simulink library "uav_library"  (R2016a)
settings: Solver=ode45  StartTime=0.0  StopTime=10.0  RelTol=1e-3
libraries: uav_library x51, aerolibutil x5, simulink x2, aerolibtransform2 x1
settings Model: Creator=Maxence  LastModifiedBy=Maxence
settings DataIOCC: LimitDataPoints=on
settings DebuggingCC: AllowSymbolicDim=off

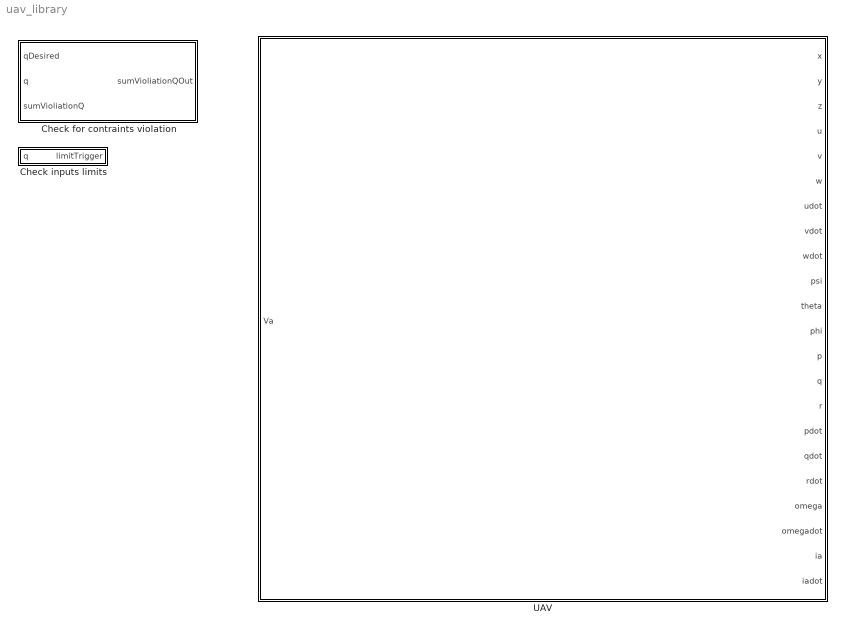
== system uav_library ==
  Check for contraints violation : Subsystem  mask{violationFactor=5, lowerQTol=0, upperQTol=0, currentTimeThreshold=0}
      mask prompts: violationFactor "Violation factor"; lowerQTol "Lower tolerance"; upperQTol "Upper tolerance"; currentTimeThreshold "Time threshold"
  Check inputs limits : Subsystem  mask{qMin=-1, qMax=1}
      mask prompts: qMin "Min value"; qMax "Max value"
  UAV : Subsystem  mask{g=9.80665, activateMast=on, config=X4, nMotors=4, m=0.312, I=[4.856e-3,0,0;0,4.856e-3,0;0,0,8.801e-3], PP=[0.16,0.16,-0.16,-0.16;0.16,-0.16,-0.16,0.16;0,0,0,0], Ra=0.5033*ones(4,1), La=1e-3*ones(4,1), ke=7.8e-3*ones(4,1), km=3.7e-3*ones(4,1), kD=1.140e-7*ones(4,1), Jm=3.357e-5*ones(4,1), Bm=1.23e-6*ones(4,1), kT=2.980e-6*ones(4,1), VaMin=0, VaMax=12, omegaInitial=zeros(4,1), omegaDelay=zeros(4,1), iaInitial=zeros(4,1), iaDelay=zeros(4,1), vPtInitial=zeros(3,1), vPtDelay=zeros(3,1), xPInitial=zeros(3,1), xPDelay=zeros(3,1), omegabtInitial=zeros(3,1), omegabtDelay=zeros(3,1), eulerZYXInitial=zeros(3,1), eulerZYXDelay=zeros(3,1)}
      mask prompts: g "Gravity (m/s^2)"; activateMast "Activate mask"; config "Configuration"; nMotors "Number of motors"; m "UAV mass (m) (kg)"; I "UAV Inertia tensor (I) (kg.m^2)"; PP "Motors position (PP) (m)"; Ra "Electrical resistance (Ra) (Ohm)"; La "Electrical inductance (La) (H)"; ke "Electromotive force constant (ke) (V/rad/s)"; km "Torque constant (km) (N.m/A)"; kD "Propeller drag parameter (kD) (N.m/rad^2/s^2)"; Jm "Rotor and propeller inertia (Jm) (kg*m^2)"; Bm "Viscous friction coefficient (Bm) (N.m/rad/s)"; kT "Propeller thrust coefficient (kT) (N/rad^2/s^2)"; VaMin "Voltage min (V)"; VaMax "Voltage max (V)"; omegaInitial "Angular velocity (rad/s)"; omegaDelay "Angular velocity delay (s)"; iaInitial "Current (A)"; iaDelay "Current delay (s)"; vPtInitial "Velocity (u, v, w) (m/s)"; vPtDelay "Velocity delay (u, v, w) (s)"; xPInitial "Position in tangent NED (m)"; xPDelay "Position in tangent NED delay (s)"; omegabtInitial "Angular rates (p, q, r) (rad/s)"; omegabtDelay "Angular rates delay (p, q, r) (s)"; eulerZYXInitial "Yaw, pitch, roll (psi, theta, phi) (rad)"; eulerZYXDelay "Yaw, pitch, roll delay (psi, theta, phi) (s)"
      mask TypeOptions config: X4 | I4 | X6 | I6 | I8 | V8
      mask Display:
      | if activateMast
      |     config = get_param(gcb,'config');
      |     position = get_param(gcb,'Position');
      |     width = abs(position(3) - position(1));
      |     height = abs(position(2) - position(4));
      |     width_ = width/1.8;
      |     if config == 'X4'
      |         height_ = width_*(654/643);
      |         posX = width/2 - width_/2;
      |         posY = height/2 - height_/2;
      |         image(imread('simulink_masks/Drone_Config_X4.jpg'),[posX,posY,width_,height_]) %
      |     elseif config == 'I4'
      |         height_ = width_*(832/850);
      |         posX = width/2 - width_/2;
      |         posY = height/2 - height_/2;
      |         image(imread('simulink_masks/Drone_Config_I4.jpg'),[posX,posY,width_,height_])
      |     elseif config == 'X6'
      |         height_ = width_*(759/811);
      |         posX = width/2 - width_/2;
      |         posY = height/2 - height_/2;
      |         image(imread('simulink_masks/Drone_Config_X6.jpg'),[posX,posY,width_,height_])
      |     elseif config == 'I6'
      |         height_ = width_*(812/732);
      |         posX = width/2 - width_/2;
      |         posY = height/2 - height_/2;
      |         image(imread('simulink_masks/Drone_Config_I6.jpg'),[posX,posY,width_,height_])
      |     elseif config == 'I8'
      |         height_ = width_*(827/809);
      |         posX = width/2 - width_/2;
      |         posY = height/2 - height_/2;
      |         image(imread('simulink_masks/Drone_Config_I8.jpg'),[posX,posY,width_,height_])
      |     elseif config == 'V8'
      |         height_ = width_*(806/784);
      |         posX = width/2 - width_/2;
      |         posY = height/2 - height_/2;
      |         image(imread('simulink_masks/Drone_Config_V8.jpg'),[posX,posY,width_,height_])
      |     end
      | end
      | 
      | % Ports label
      | port_label('input', 1, 'Va (V)')
      | port_label('output', 1, 'x (m)')
      | port_label('output', 2, 'y (m)')
      | port_label('output', 3, 'z (m)')
      | port_label('output', 4, 'u (m/s)')
      | port_label('output', 5, 'v (m/s)')
      | port_label('output', 6, 'w (m/s)')
      | port_label('output', 7, 'du/dt (m/s^2)')
      | port_label('output', 8, 'dv/dt (m/s^2)')
      | port_label('output', 9, 'dw/dt (m/s^2)')
      | port_label('output', 10, 'psi (rad)')
      | port_label('output', 11, 'theta (rad)')
      | port_label('output', 12, 'phi (rad)')
      | port_label('output', 13, 'p (rad/s)')
      | port_label('output', 14, 'q (rad/s)')
      | port_label('output', 15, 'r (rad/s)')
      | port_label('output', 16, 'dp/dt (rad/s^2)')
      | port_label('output', 17, 'dq/dt (rad/s^2)')
      | port_label('output', 18, 'dr/dt (rad/s^2)')
      | port_label('output', 19, 'omega (rad/s)')
      | port_label('output', 20, 'domega/dt (rad/s^2)')
      | port_label('output', 21, 'ia (A)')
      | port_label('output', 22, 'dia/dt (A/s)')

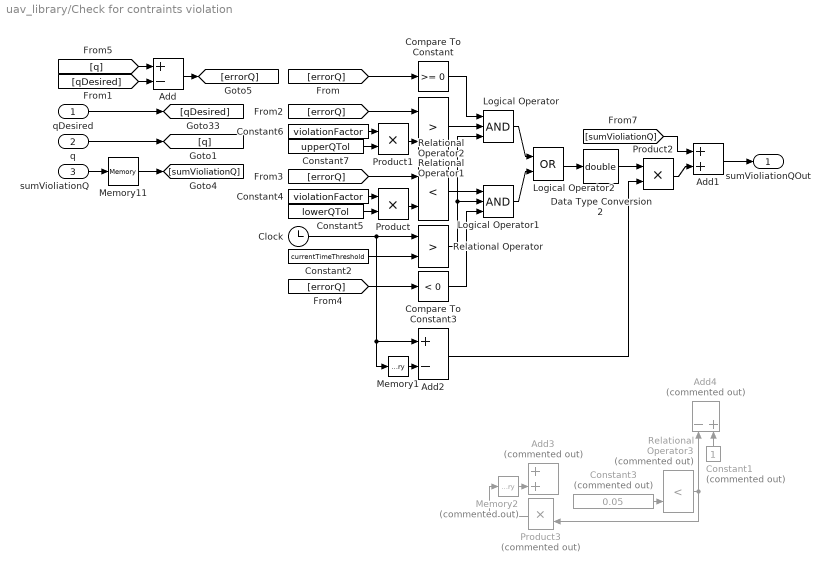
== system uav_library/Check for contraints violation ==
  qDesired : Inport
  q : Inport  Port=2
  sumVioliationQ : Inport  Port=3
  Add : Sum  Inputs=+-
  Add1 : Sum
  Add2 : Sum  Inputs=+-
  Add3 : Sum  Commented=on
  Add4 : Sum  Commented=on  Inputs=-+
  Clock : Clock
  Compare To Constant : simulink/Logic and Bit Operations/Compare To Constant  relop=>=  const=0  OutDataTypeStr=boolean  ZeroCross=off
  Compare To Constant3 : simulink/Logic and Bit Operations/Compare To Constant  relop=<  const=0  OutDataTypeStr=boolean  ZeroCross=off
  Constant1 : Constant  Commented=on
  Constant2 : Constant  Value=currentTimeThreshold
  Constant3 : Constant  Commented=on  Value=0.05
  Constant4 : Constant  Value=violationFactor
  Constant5 : Constant  Value=lowerQTol
  Constant6 : Constant  Value=violationFactor
  Constant7 : Constant  Value=upperQTol
  Data Type Conversion2 : DataTypeConversion  OutDataTypeStr=double
  Logical Operator : Logic  Inputs=3  AllPortsSameDT=off  OutDataTypeStr=boolean
  Logical Operator1 : Logic  Inputs=3  AllPortsSameDT=off  OutDataTypeStr=boolean
  Logical Operator2 : Logic  Operator=OR  AllPortsSameDT=off  OutDataTypeStr=boolean
  Memory1 : Memory
  Memory11 : Memory
  Memory2 : Memory  Commented=on
  Product : Product
  Product1 : Product
  Product2 : Product
  Product3 : Product  Commented=on
  Relational Operator : RelationalOperator  Operator=>  OutDataTypeStr=boolean  ZeroCross=off
  Relational Operator1 : RelationalOperator  Operator=>  OutDataTypeStr=boolean  ZeroCross=off
  Relational Operator2 : RelationalOperator  Operator=<  OutDataTypeStr=boolean  ZeroCross=off
  Relational Operator3 : RelationalOperator  Commented=on  Operator=<  OutDataTypeStr=boolean  ZeroCross=off
  sumVioliationQOut : Outport
  wires:
  qDesired/1 -> [qDesired]
  q/1 -> [q]
  sumVioliationQ/1 -> Memory11/1
  [q] -> Add/1
  [qDesired] -> Add/2
  Add/1 -> [errorQ]
  [errorQ] -> Compare To Constant/1
  Constant2/1 -> Relational Operator/2
  Constant4/1 -> Product/1
  Constant5/1 -> Product/2
  Constant6/1 -> Product1/1
  Constant7/1 -> Product1/2
  [errorQ] -> Relational Operator1/1
  Product1/1 -> Relational Operator1/2
  [errorQ] -> Relational Operator2/1
  Product/1 -> Relational Operator2/2
  Relational Operator2/1 -> Logical Operator1/1
  Relational Operator1/1 -> Logical Operator/2
  Relational Operator/1 -> Logical Operator/3, Logical Operator1/2
  [errorQ] -> Compare To Constant3/1
  Compare To Constant3/1 -> Logical Operator1/3
  Compare To Constant/1 -> Logical Operator/1
  Add1/1 -> sumVioliationQOut/1
  [sumVioliationQ] -> Add1/1
  Logical Operator/1 -> Logical Operator2/1
  Logical Operator1/1 -> Logical Operator2/2
  Logical Operator2/1 -> Data Type Conversion2/1
  Memory11/1 -> [sumVioliationQ]
  Data Type Conversion2/1 -> Product2/1
  Product2/1 -> Add1/2
  Clock/1 -> Relational Operator/1, Memory1/1, Add2/1
  Memory1/1 -> Add2/2
  Add2/1 -> Product2/2
  Memory2/1 -> Add3/2
  Constant3/1 -> Relational Operator3/2
  Product3/1 -> Memory2/1
  Relational Operator3/1 -> Add4/1, Product3/2
  Constant1/1 -> Add4/2

== system uav_library/Check inputs limits ==
  q : Inport
  Constant5 : Constant  Value=qMin
  Constant6 : Constant  Value=qMax
  Data Type Conversion2 : DataTypeConversion  OutDataTypeStr=double
  Logical Operator2 : Logic  Operator=OR  AllPortsSameDT=off  OutDataTypeStr=boolean
  Relational Operator12 : RelationalOperator  Operator=<  OutDataTypeStr=boolean  ZeroCross=off
  Relational Operator13 : RelationalOperator  Operator=>  OutDataTypeStr=boolean  ZeroCross=off
  limitTrigger : Outport
  wires:
  Constant5/1 -> Relational Operator12/2
  Constant6/1 -> Relational Operator13/2
  q/1 -> Relational Operator13/1, Relational Operator12/1
  Relational Operator12/1 -> Logical Operator2/1
  Relational Operator13/1 -> Logical Operator2/2
  Logical Operator2/1 -> Data Type Conversion2/1
  Data Type Conversion2/1 -> limitTrigger/1

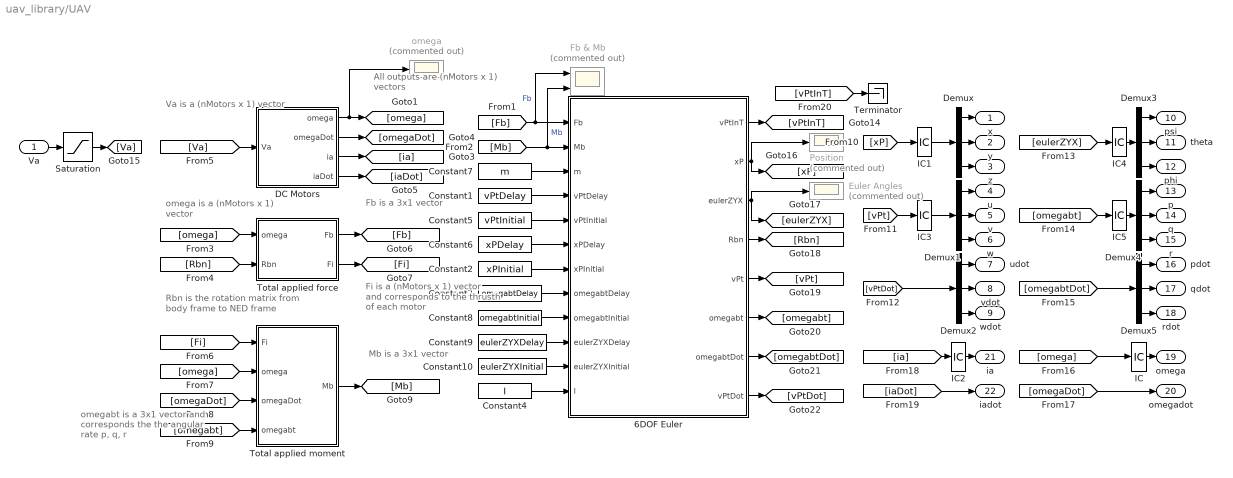
== system uav_library/UAV ==
  note: Va is a (nMotors x 1) vector
  note: All outputs are (nMotors x 1) vectors
  note: Rbn is the rotation matrix from body frame to NED frame
  note: omega is a (nMotors x 1) vector
  note: Fb is a 3x1 vector
  note: Fi is a (nMotors x 1) vector and corresponds to the thrusth of each motor
  note: Mb is a 3x1 vector
  note: omegabt is a 3x1 vector and corresponds the the angular rate p, q, r
  Va : Inport
  " omega" : Scope  Commented=on
  6DOF Euler : Subsystem
  Constant1 : Constant  Value=vPtDelay
  Constant10 : Constant  Value=eulerZYXInitial
  Constant2 : Constant  Value=xPInitial
  Constant3 : Constant  Value=omegabtDelay
  Constant4 : Constant  Value=I
  Constant5 : Constant  Value=vPtInitial
  Constant6 : Constant  Value=xPDelay
  Constant7 : Constant  Value=m
  Constant8 : Constant  Value=omegabtInitial
  Constant9 : Constant  Value=eulerZYXDelay
  DC Motors : Subsystem
  Demux{,1..5} (6 alike) : Demux  Outputs=3
  Euler Angles : Scope  Commented=on
  Fb & Mb : Scope  Commented=on  NumInputPorts=2
  IC : InitialCondition  Value=omegaInitial
  IC1 : InitialCondition  Value=xPInitial
  IC2 : InitialCondition  Value=iaInitial
  IC3 : InitialCondition  Value=vPtInitial
  IC4 : InitialCondition  Value=eulerZYXInitial
  IC5 : InitialCondition  Value=omegabtInitial
  Position : Scope  Commented=on
  Saturation : Saturate  UpperLimit=VaMax  LowerLimit=VaMin
  Terminator : Terminator
  Total applied force : Subsystem
  Total applied moment : Subsystem
  x : Outport
  y : Outport  Port=2
  z : Outport  Port=3
  u : Outport  Port=4
  v : Outport  Port=5
  w : Outport  Port=6
  udot : Outport  Port=7
  vdot : Outport  Port=8
  wdot : Outport  Port=9
  psi : Outport  Port=10
  theta : Outport  Port=11
  phi : Outport  Port=12
  p : Outport  Port=13
  q : Outport  Port=14
  r : Outport  Port=15
  pdot : Outport  Port=16
  qdot : Outport  Port=17
  rdot : Outport  Port=18
  omega : Outport  Port=19
  omegadot : Outport  Port=20
  ia : Outport  Port=21
  iadot : Outport  Port=22
  wires:
  DC Motors/1(omega) -> " omega"/1, [omega]
  DC Motors/3(ia) -> [ia]
  DC Motors/2(omegaDot) -> [omegaDot]
  DC Motors/4(iaDot) -> [iaDot]
  Total applied force/1(Fb) -> [Fb]
  [Fb] -> 6DOF Euler/1(Fb), Fb & Mb/1  "Fb"
  [Mb] -> 6DOF Euler/2(Mb), Fb & Mb/2  "Mb"
  [omega] -> Total applied force/1(omega)
  [Rbn] -> Total applied force/2(Rbn)
  Total applied force/2(Fi) -> [Fi]
  [Va] -> DC Motors/1(Va)
  [Fi] -> Total applied moment/1(Fi)
  [omega] -> Total applied moment/2(omega)
  [omegaDot] -> Total applied moment/3(omegaDot)
  [omegabt] -> Total applied moment/4(omegabt)
  Total applied moment/1(Mb) -> [Mb]
  6DOF Euler/1(vPtInT) -> [vPtInT]
  [xP] -> IC1/1
  Demux/1 -> x/1
  Demux/2 -> y/1
  Demux/3 -> z/1
  6DOF Euler/2(xP) -> Position/1, [xP]
  6DOF Euler/3(eulerZYX) -> Euler Angles/1, [eulerZYX]
  6DOF Euler/4(Rbn) -> [Rbn]
  6DOF Euler/5(vPt) -> [vPt]
  6DOF Euler/6(omegabt) -> [omegabt]
  6DOF Euler/7(omegabtDot) -> [omegabtDot]
  6DOF Euler/8(vPtDot) -> [vPtDot]
  Constant7/1 -> 6DOF Euler/3(m)
  Constant1/1 -> 6DOF Euler/4(vPtDelay)
  Constant4/1 -> 6DOF Euler/12(I)
  Constant5/1 -> 6DOF Euler/5(vPtInitial)
  Constant6/1 -> 6DOF Euler/6(xPDelay)
  Constant2/1 -> 6DOF Euler/7(xPInitial)
  Constant3/1 -> 6DOF Euler/8(omegabtDelay)
  Constant8/1 -> 6DOF Euler/9(omegabtInitial)
  Constant9/1 -> 6DOF Euler/10(eulerZYXDelay)
  Constant10/1 -> 6DOF Euler/11(eulerZYXInitial)
  Va/1 -> Saturation/1
  [vPt] -> IC3/1
  Demux1/1 -> u/1
  Demux1/2 -> v/1
  Demux1/3 -> w/1
  [vPtDot] -> Demux2/1
  Demux2/1 -> udot/1
  Demux2/2 -> vdot/1
  Demux2/3 -> wdot/1
  [eulerZYX] -> IC4/1
  Demux3/1 -> psi/1
  Demux3/2 -> theta/1
  Demux3/3 -> phi/1
  Demux4/1 -> p/1
  Demux4/2 -> q/1
  Demux4/3 -> r/1
  [omegabtDot] -> Demux5/1
  Demux5/1 -> pdot/1
  Demux5/2 -> qdot/1
  Demux5/3 -> rdot/1
  [omega] -> IC/1
  [ia] -> IC2/1
  Saturation/1 -> [Va]
  [vPtInT] -> Terminator/1
  IC/1 -> omega/1
  [omegaDot] -> omegadot/1
  IC2/1 -> ia/1
  [iaDot] -> iadot/1
  IC1/1 -> Demux/1
  IC3/1 -> Demux1/1
  IC4/1 -> Demux3/1
  [omegabt] -> IC5/1
  IC5/1 -> Demux4/1

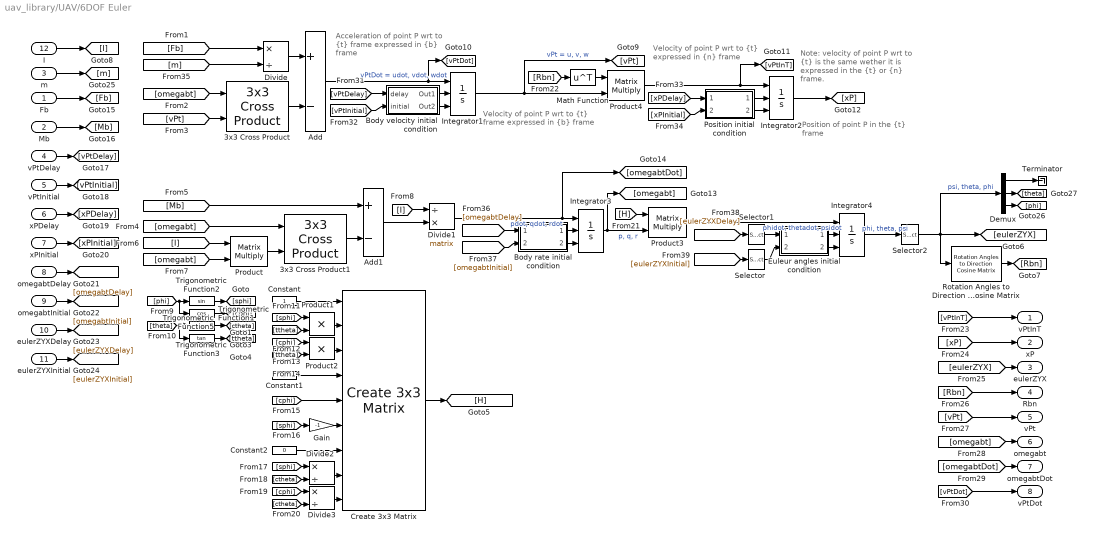
== system uav_library/UAV/6DOF Euler ==
  note: Acceleration of point P wrt to {t} frame expressed in {b} frame
  note: Velocity of point P wrt to {t} frame expressed in {b} frame
  note: Velocity of point P wrt to {t} expressed in {n} frame
  note: Position of point P in the {t} frame
  note: Note: velocity of point P wrt to {t} is the same wether it is expressed in the {t} or {n} frame.
  Fb : Inport
  Mb : Inport  Port=2
  m : Inport  Port=3
  vPtDelay : Inport  Port=4
  vPtInitial : Inport  Port=5
  xPDelay : Inport  Port=6
  xPInitial : Inport  Port=7
  omegabtDelay : Inport  Port=8
  omegabtInitial : Inport  Port=9
  eulerZYXDelay : Inport  Port=10
  eulerZYXInitial : Inport  Port=11
  I : Inport  Port=12
  3x3 Cross Product : aerolibutil/3x3 Cross Product
  3x3 Cross Product1 : aerolibutil/3x3 Cross Product
  Add : Sum  Inputs=+-
  Add1 : Sum  Inputs=+-
  Body rate initial condition : Subsystem
  Body velocity initial condition : Subsystem
  Constant : Constant
  Constant1 : Constant  Value=0
  Constant2 : Constant  Value=0
  Create 3x3 Matrix : aerolibutil/Create 3x3 Matrix
  Demux : Demux  Outputs=3
  Divide : Product  Inputs=*/
  Divide1 : Product  Inputs=/*  Multiplication=Matrix(*)
  Divide2 : Product  Inputs=*/
  Divide3 : Product  Inputs=*/
  Euleur angles initial condition : Subsystem
  Gain : Gain  Gain=-1
  Integrator1 : Integrator  ExternalReset=falling  InitialConditionSource=external
  Integrator2 : Integrator  ExternalReset=falling  InitialConditionSource=external
  Integrator3 : Integrator  ExternalReset=falling  InitialConditionSource=external
  Integrator4 : Integrator  ExternalReset=falling  InitialConditionSource=external  WrapState=on  WrappedStateUpperValue=[pi;pi/2;pi]  WrappedStateLowerValue=-[pi;pi/2;pi]
  Math Function : Math  Operator=transpose  SaturateOnIntegerOverflow=on
  Position initial condition : Subsystem
  Product : Product  Multiplication=Matrix(*)
  Product1 : Product
  Product2 : Product
  Product3 : Product  Multiplication=Matrix(*)
  Product4 : Product  Multiplication=Matrix(*)
  Rotation Angles to Direction Cosine Matrix : aerolibtransform2/Rotation Angles to Direction Cosine Matrix  rotationOrder=ZYX
  Selector : Selector  InputPortWidth=3  IndexOptions=Index vector (dialog)  Indices=[3 2 1]  OutputSizes=1
  Selector1 : Selector  InputPortWidth=3  IndexOptions=Index vector (dialog)  Indices=[3 2 1]  OutputSizes=1
  Selector2 : Selector  InputPortWidth=3  IndexOptions=Index vector (dialog)  Indices=[3 2 1]  OutputSizes=1
  Terminator : Terminator
  Trigonometric Function1 : Trigonometry  Operator=cos
  Trigonometric Function2 : Trigonometry
  Trigonometric Function3 : Trigonometry  Operator=cos
  Trigonometric Function5 : Trigonometry  Operator=tan
  vPtInT : Outport
  xP : Outport  Port=2
  eulerZYX : Outport  Port=3
  Rbn : Outport  Port=4
  vPt : Outport  Port=5
  omegabt : Outport  Port=6
  omegabtDot : Outport  Port=7
  vPtDot : Outport  Port=8
  wires:
  [omegabt] -> 3x3 Cross Product/1
  [vPt] -> 3x3 Cross Product/2
  [m] -> Divide/2
  [Fb] -> Divide/1
  Divide/1 -> Add/1
  3x3 Cross Product/1 -> Add/2
  Add/1 -> [vPtDot], Integrator1/1  "vPtDot = udot, vdot, wdot"
  Body velocity initial condition/1(Out1) -> Integrator1/2
  Body velocity initial condition/2(Out2) -> Integrator1/3
  [vPtDelay] -> Body velocity initial condition/1(delay)
  [vPtInitial] -> Body velocity initial condition/2(initial)
  Integrator1/1 -> Product4/2, [vPt]  "vPt = u, v, w"
  Position initial condition/1(Out1) -> Integrator2/2
  Position initial condition/2(Out2) -> Integrator2/3
  [xPDelay] -> Position initial condition/1(delay)
  [xPInitial] -> Position initial condition/2(initial)
  [omegabt] -> 3x3 Cross Product1/1
  [I] -> Product/1
  [omegabt] -> Product/2
  Product/1 -> 3x3 Cross Product1/2
  [Mb] -> Add1/1
  3x3 Cross Product1/1 -> Add1/2
  [I] -> Divide1/1
  Add1/1 -> Divide1/2
  Body rate initial condition/1(Out1) -> Integrator3/2
  Body rate initial condition/2(Out2) -> Integrator3/3
  [omegabtDelay] -> Body rate initial condition/1(delay)
  [omegabtInitial] -> Body rate initial condition/2(initial)
  Divide1/1 -> [omegabtDot], Integrator3/1  "pdot, qdot, rdot"
  Constant/1 -> Create 3x3 Matrix/1
  Constant1/1 -> Create 3x3 Matrix/4
  Constant2/1 -> Create 3x3 Matrix/7
  [phi] -> Trigonometric Function1/1, Trigonometric Function2/1
  Trigonometric Function2/1 -> [sphi]
  Trigonometric Function1/1 -> [cphi]
  [theta] -> Trigonometric Function5/1, Trigonometric Function3/1
  Trigonometric Function3/1 -> [ctheta]
  Trigonometric Function5/1 -> [ttheta]
  Product1/1 -> Create 3x3 Matrix/2
  [sphi] -> Product1/1
  [ttheta] -> Product1/2
  [cphi] -> Product2/1
  [ttheta] -> Product2/2
  Product2/1 -> Create 3x3 Matrix/3
  [cphi] -> Create 3x3 Matrix/5
  [sphi] -> Gain/1
  Gain/1 -> Create 3x3 Matrix/6
  Divide2/1 -> Create 3x3 Matrix/8
  Divide3/1 -> Create 3x3 Matrix/9
  [sphi] -> Divide2/1
  [ctheta] -> Divide2/2
  [cphi] -> Divide3/1
  [ctheta] -> Divide3/2
  Create 3x3 Matrix/1 -> [H]
  Integrator3/1 -> [omegabt], Product3/2  "p, q, r"
  [H] -> Product3/1
  Product3/1 -> Integrator4/1  "phidot, thetadot, psidot"
  Euleur angles initial condition/1(Out1) -> Integrator4/2
  Euleur angles initial condition/2(Out2) -> Integrator4/3
  Integrator4/1 -> Selector2/1  "phi, theta, psi"
  [eulerZYXInitial] -> Selector/1
  [eulerZYXDelay] -> Selector1/1
  Selector1/1 -> Euleur angles initial condition/1(delay)
  Selector/1 -> Euleur angles initial condition/2(initial)
  Selector2/1 -> Demux/1, Rotation Angles to Direction Cosine Matrix/1, [eulerZYX]  "psi, theta, phi"
  Rotation Angles to Direction Cosine Matrix/1 -> [Rbn]
  [Rbn] -> Math Function/1
  Product4/1 -> [vPtInT], Integrator2/1
  Integrator2/1 -> [xP]
  [vPtInT] -> vPtInT/1
  [xP] -> xP/1
  [eulerZYX] -> eulerZYX/1
  [Rbn] -> Rbn/1
  [vPt] -> vPt/1
  [omegabt] -> omegabt/1
  [omegabtDot] -> omegabtDot/1
  [vPtDot] -> vPtDot/1
  Fb/1 -> [Fb]
  Mb/1 -> [Mb]
  vPtDelay/1 -> [vPtDelay]
  vPtInitial/1 -> [vPtInitial]
  xPDelay/1 -> [xPDelay]
  xPInitial/1 -> [xPInitial]
  omegabtDelay/1 -> [omegabtDelay]
  omegabtInitial/1 -> [omegabtInitial]
  eulerZYXDelay/1 -> [eulerZYXDelay]
  eulerZYXInitial/1 -> [eulerZYXInitial]
  m/1 -> [m]
  Demux/2 -> [theta]
  Demux/3 -> [phi]
  Demux/1 -> Terminator/1
  I/1 -> [I]
  Math Function/1 -> Product4/1

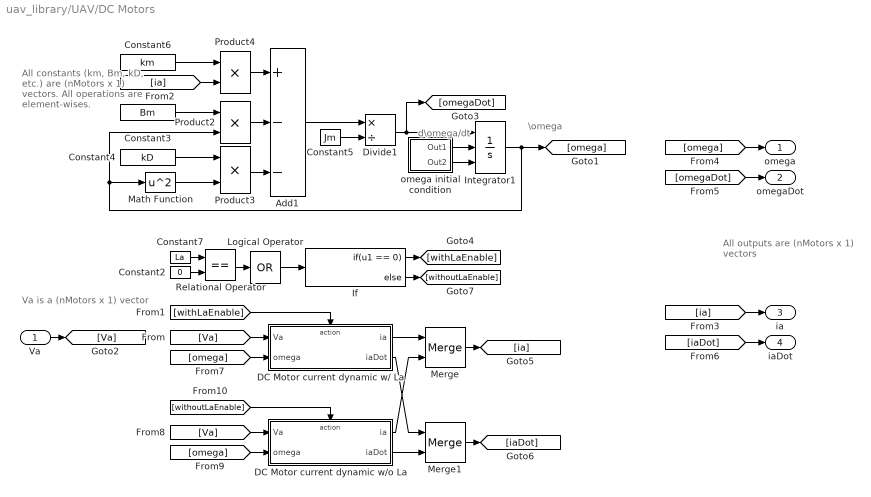
== system uav_library/UAV/DC Motors ==
  note: d\omega/dt
  note: \omega
  note: Va is a (nMotors x 1) vector
  note: All constants (km, Bm, kD, etc.) are (nMotors x 1) vectors.
      |
      | All operations are element-wises.
  note: All outputs are (nMotors x 1) vectors
  Va : Inport
  Add1 : Sum  Inputs=+--
  Constant2 : Constant  Value=0
  Constant3 : Constant  Value=Bm
  Constant4 : Constant  Value=kD
  Constant5 : Constant  Value=Jm
  Constant6 : Constant  Value=km
  Constant7 : Constant  Value=La
  DC Motor current dynamic w/ La : Subsystem  TreatAsAtomicUnit=on
  DC Motor current dynamic w/o La : Subsystem  TreatAsAtomicUnit=on
  Divide1 : Product  Inputs=*/
  If : If  IfExpression=u1 == 0
  Integrator1 : Integrator  ExternalReset=falling  InitialConditionSource=external
  Logical Operator : Logic  Operator=OR  Inputs=1  AllPortsSameDT=off  OutDataTypeStr=boolean
  Math Function : Math  Operator=square  SaturateOnIntegerOverflow=on
  Merge : Merge
  Merge1 : Merge
  Product2 : Product
  Product3 : Product
  Product4 : Product
  Relational Operator : RelationalOperator  Operator===  OutDataTypeStr=boolean
  omega initial condition : Subsystem
  omega : Outport
  omegaDot : Outport  Port=2
  ia : Outport  Port=3
  iaDot : Outport  Port=4
  wires:
  Product4/1 -> Add1/1
  Constant6/1 -> Product4/1
  [ia] -> Product4/2
  Product2/1 -> Add1/2
  Integrator1/1 -> [omega], Math Function/1, Product2/2
  Add1/1 -> Divide1/1
  Constant4/1 -> Product3/1
  Constant3/1 -> Product2/1
  Product3/1 -> Add1/3
  Constant5/1 -> Divide1/2
  Math Function/1 -> Product3/2
  Va/1 -> [Va]
  [ia] -> ia/1
  [omega] -> omega/1
  [omegaDot] -> omegaDot/1
  [iaDot] -> iaDot/1
  Divide1/1 -> [omegaDot], Integrator1/1
  omega initial condition/1(Out1) -> Integrator1/2
  omega initial condition/2(Out2) -> Integrator1/3
  Logical Operator/1 -> If/1
  DC Motor current dynamic w/o La/2(iaDot) -> Merge1/2
  [Va] -> DC Motor current dynamic w/ La/1(Va)
  DC Motor current dynamic w/ La/1(ia) -> Merge/1
  Merge/1 -> [ia]
  Merge1/1 -> [iaDot]
  [omega] -> DC Motor current dynamic w/ La/2(omega)
  [omega] -> DC Motor current dynamic w/o La/2(omega)
  [Va] -> DC Motor current dynamic w/o La/1(Va)
  If/1 -> [withLaEnable]
  If/2 -> [withoutLaEnable]
  [withLaEnable] -> DC Motor current dynamic w/ La/Action
  [withoutLaEnable] -> DC Motor current dynamic w/o La/Action
  DC Motor current dynamic w/ La/2(iaDot) -> Merge1/1
  DC Motor current dynamic w/o La/1(ia) -> Merge/2
  Relational Operator/1 -> Logical Operator/1
  Constant2/1 -> Relational Operator/2
  Constant7/1 -> Relational Operator/1

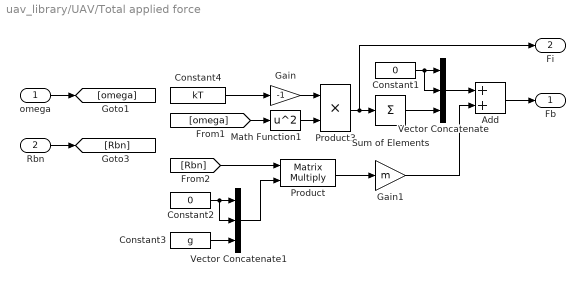
== system uav_library/UAV/Total applied force ==
  omega : Inport
  Rbn : Inport  Port=2
  Add : Sum
  Constant1 : Constant  Value=0
  Constant2 : Constant  Value=0
  Constant3 : Constant  Value=g
  Constant4 : Constant  Value=kT
  Gain : Gain  Gain=-1
  Gain1 : Gain  Gain=m
  Math Function1 : Math  Operator=square  SaturateOnIntegerOverflow=on
  Product : Product  Multiplication=Matrix(*)
  Product3 : Product
  Sum of Elements : Sum  Inputs=+
  Vector Concatenate : Concatenate  NumInputs=3
  Vector Concatenate1 : Concatenate  NumInputs=3
  Fb : Outport
  Fi : Outport  Port=2
  wires:
  Constant4/1 -> Gain/1
  Math Function1/1 -> Product3/2
  Product/1 -> Gain1/1
  Constant2/1 -> Vector Concatenate1/2, Vector Concatenate1/1
  Constant3/1 -> Vector Concatenate1/3
  Product3/1 -> Fi/1, Sum of Elements/1
  Add/1 -> Fb/1
  Vector Concatenate1/1 -> Product/2
  Sum of Elements/1 -> Vector Concatenate/3
  Gain/1 -> Product3/1
  Constant1/1 -> Vector Concatenate/2, Vector Concatenate/1
  Vector Concatenate/1 -> Add/1
  [omega] -> Math Function1/1
  omega/1 -> [omega]
  Rbn/1 -> [Rbn]
  [Rbn] -> Product/1
  Gain1/1 -> Add/2

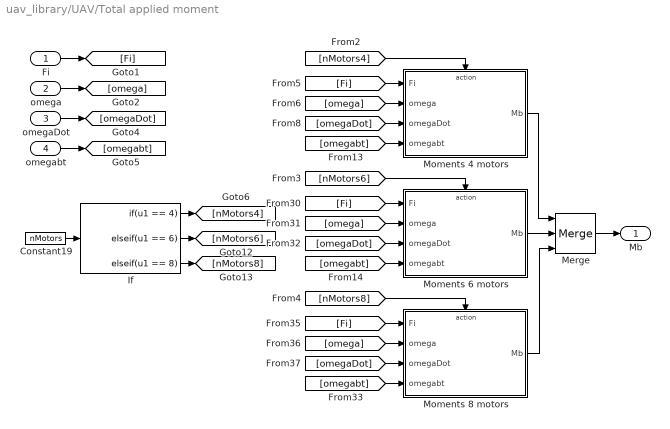
== system uav_library/UAV/Total applied moment ==
  Fi : Inport
  omega : Inport  Port=2
  omegaDot : Inport  Port=3
  omegabt : Inport  Port=4
  Constant19 : Constant  Value=nMotors
  If : If  IfExpression=u1 == 4  ElseIfExpressions=u1 == 6, u1 == 8  ShowElse=off
  Merge : Merge  Inputs=3
  Moments 4 motors : Subsystem  TreatAsAtomicUnit=on
  Moments 6 motors : Subsystem  TreatAsAtomicUnit=on
  Moments 8 motors : Subsystem  TreatAsAtomicUnit=on
  Mb : Outport
  wires:
  Fi/1 -> [Fi]
  omega/1 -> [omega]
  omegaDot/1 -> [omegaDot]
  omegabt/1 -> [omegabt]
  If/1 -> [nMotors4]
  If/2 -> [nMotors6]
  [nMotors4] -> Moments 4 motors/Action
  [nMotors6] -> Moments 6 motors/Action
  Constant19/1 -> If/1
  If/3 -> [nMotors8]
  [Fi] -> Moments 4 motors/1(Fi)
  [omega] -> Moments 4 motors/2(omega)
  [omegaDot] -> Moments 4 motors/3(omegaDot)
  [omegabt] -> Moments 4 motors/4(omegabt)
  [Fi] -> Moments 6 motors/1(Fi)
  [omega] -> Moments 6 motors/2(omega)
  [omegaDot] -> Moments 6 motors/3(omegaDot)
  [omegabt] -> Moments 6 motors/4(omegabt)
  [nMotors8] -> Moments 8 motors/Action
  [Fi] -> Moments 8 motors/1(Fi)
  [omega] -> Moments 8 motors/2(omega)
  [omegaDot] -> Moments 8 motors/3(omegaDot)
  [omegabt] -> Moments 8 motors/4(omegabt)
  Moments 6 motors/1(Mb) -> Merge/2
  Moments 4 motors/1(Mb) -> Merge/1
  Moments 8 motors/1(Mb) -> Merge/3
  Merge/1 -> Mb/1

== system uav_library/UAV/6DOF Euler/Body rate initial condition ==
  delay : Inport
  initial : Inport  Port=2
  Clock1 : Clock
  Sum4 : Sum  Inputs=|-+
  Triggered Subsystem2 : Subsystem  TreatAsAtomicUnit=on
  Out1 : Outport
  Out2 : Outport  Port=2
  wires:
  delay/1 -> Sum4/2
  Triggered Subsystem2/1(Out1) -> Out2/1
  Sum4/1 -> Out1/1, Triggered Subsystem2/Trigger
  Clock1/1 -> Sum4/1
  initial/1 -> Triggered Subsystem2/1(In1)

== system uav_library/UAV/6DOF Euler/Body velocity initial condition ==
  delay : Inport
  initial : Inport  Port=2
  Clock1 : Clock
  Sum4 : Sum  Inputs=|-+
  Triggered Subsystem2 : Subsystem  TreatAsAtomicUnit=on
  Out1 : Outport
  Out2 : Outport  Port=2
  wires:
  delay/1 -> Sum4/2
  Triggered Subsystem2/1(Out1) -> Out2/1
  Sum4/1 -> Out1/1, Triggered Subsystem2/Trigger
  Clock1/1 -> Sum4/1
  initial/1 -> Triggered Subsystem2/1(In1)

== system uav_library/UAV/6DOF Euler/Euleur angles initial condition ==
  delay : Inport
  initial : Inport  Port=2
  Clock1 : Clock
  Sum4 : Sum  Inputs=|-+
  Triggered Subsystem2 : Subsystem  TreatAsAtomicUnit=on
  Out1 : Outport
  Out2 : Outport  Port=2
  wires:
  delay/1 -> Sum4/2
  Triggered Subsystem2/1(Out1) -> Out2/1
  Sum4/1 -> Out1/1, Triggered Subsystem2/Trigger
  Clock1/1 -> Sum4/1
  initial/1 -> Triggered Subsystem2/1(In1)

== system uav_library/UAV/6DOF Euler/Position initial condition ==
  delay : Inport
  initial : Inport  Port=2
  Clock1 : Clock
  Sum4 : Sum  Inputs=|-+
  Triggered Subsystem2 : Subsystem  TreatAsAtomicUnit=on
  Out1 : Outport
  Out2 : Outport  Port=2
  wires:
  initial/1 -> Triggered Subsystem2/1(In1)
  Clock1/1 -> Sum4/1
  Sum4/1 -> Triggered Subsystem2/Trigger, Out1/1
  Triggered Subsystem2/1(Out1) -> Out2/1
  delay/1 -> Sum4/2

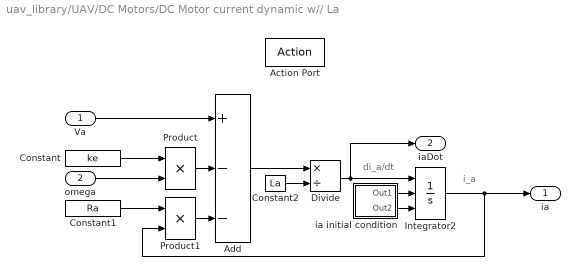
== system uav_library/UAV/DC Motors/DC Motor current dynamic w// La ==
  note: di_a/dt
  note: i_a
  Va : Inport
  omega : Inport  Port=2
  Action Port : ActionPort
  Add : Sum  Inputs=+--
  Constant : Constant  Value=ke
  Constant1 : Constant  Value=Ra
  Constant2 : Constant  Value=La
  Divide : Product  Inputs=*/
  Integrator2 : Integrator  ExternalReset=falling  InitialConditionSource=external
  Product : Product
  Product1 : Product
  ia initial condition : Subsystem
  ia : Outport
  iaDot : Outport  Port=2
  wires:
  Va/1 -> Add/1
  Product/1 -> Add/2
  Divide/1 -> iaDot/1, Integrator2/1
  Constant1/1 -> Product1/1
  Integrator2/1 -> ia/1, Product1/2
  omega/1 -> Product/2
  Add/1 -> Divide/1
  Product1/1 -> Add/3
  Constant2/1 -> Divide/2
  Constant/1 -> Product/1
  ia initial condition/1(Out1) -> Integrator2/2
  ia initial condition/2(Out2) -> Integrator2/3

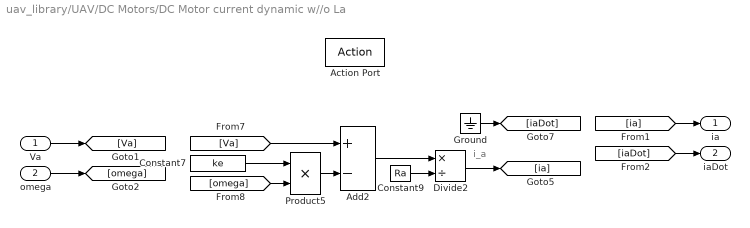
== system uav_library/UAV/DC Motors/DC Motor current dynamic w//o La ==
  note: i_a
  Va : Inport
  omega : Inport  Port=2
  Action Port : ActionPort
  Add2 : Sum  Inputs=+-
  Constant7 : Constant  Value=ke
  Constant9 : Constant  Value=Ra
  Divide2 : Product  Inputs=*/
  Ground : Ground
  Product5 : Product
  ia : Outport
  iaDot : Outport  Port=2
  wires:
  [omega] -> Product5/2
  [Va] -> Add2/1
  Divide2/1 -> [ia]
  Add2/1 -> Divide2/1
  Product5/1 -> Add2/2
  Constant9/1 -> Divide2/2
  Constant7/1 -> Product5/1
  Ground/1 -> [iaDot]
  Va/1 -> [Va]
  omega/1 -> [omega]
  [ia] -> ia/1
  [iaDot] -> iaDot/1

== system uav_library/UAV/DC Motors/omega initial condition ==
  Clock1 : Clock
  Constant3 : Constant  Value=omegaInitial
  Constant6 : Constant  Value=omegaDelay
  Sum4 : Sum  Inputs=|-+
  Triggered Subsystem2 : Subsystem  TreatAsAtomicUnit=on
  Out1 : Outport
  Out2 : Outport  Port=2
  wires:
  Constant6/1 -> Sum4/2
  Triggered Subsystem2/1(Out1) -> Out2/1
  Sum4/1 -> Out1/1, Triggered Subsystem2/Trigger
  Clock1/1 -> Sum4/1
  Constant3/1 -> Triggered Subsystem2/1(In1)

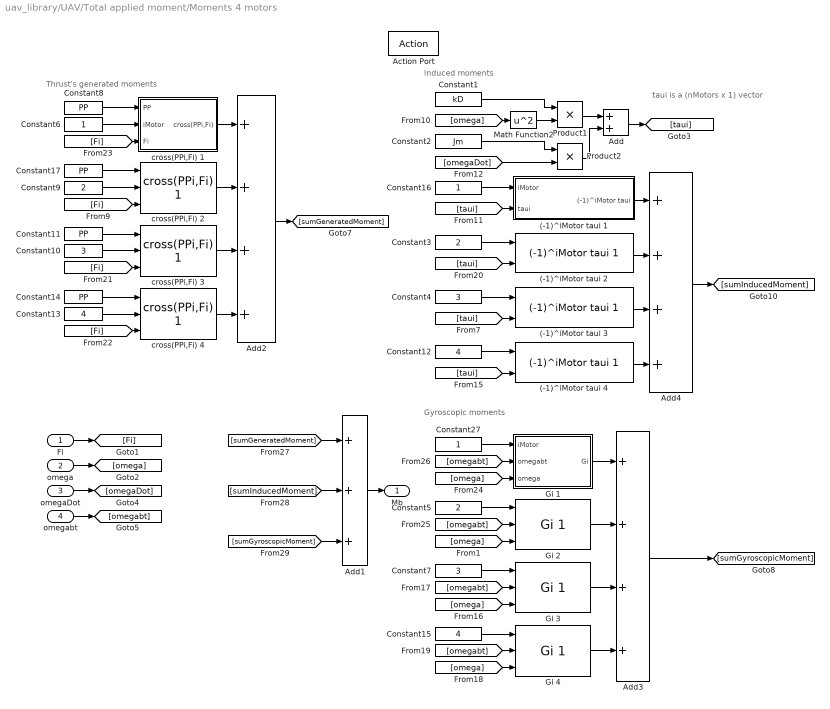
== system uav_library/UAV/Total applied moment/Moments 4 motors ==
  note: taui is a (nMotors x 1) vector
  note: Induced moments
  note: Gyroscopic moments
  note: Thrust's generated moments
  Fi : Inport
  omega : Inport  Port=2
  omegaDot : Inport  Port=3
  omegabt : Inport  Port=4
  Action Port : ActionPort
  (-1)^iMotor taui 1 : Subsystem
  (-1)^iMotor taui 2 : uav_library/UAV/Total applied moment/Moments 4 motors/(-1)^iMotor taui 1
  (-1)^iMotor taui 3 : uav_library/UAV/Total applied moment/Moments 4 motors/(-1)^iMotor taui 1
  (-1)^iMotor taui 4 : uav_library/UAV/Total applied moment/Moments 4 motors/(-1)^iMotor taui 1
  Add : Sum
  Add1 : Sum  Inputs=+++
  Add2 : Sum  Inputs=++++
  Add3 : Sum  Inputs=++++
  Add4 : Sum  Inputs=++++
  Constant1 : Constant  Value=kD
  Constant10 : Constant  Value=3
  Constant{8,11,14,17} (4 alike) : Constant  Value=PP
  Constant12 : Constant  Value=4
  Constant13 : Constant  Value=4
  Constant15 : Constant  Value=4
  Constant16 : Constant
  Constant2 : Constant  Value=Jm
  Constant27 : Constant
  Constant3 : Constant  Value=2
  Constant4 : Constant  Value=3
  Constant5 : Constant  Value=2
  Constant6 : Constant
  Constant7 : Constant  Value=3
  Constant9 : Constant  Value=2
  Gi 1 : Subsystem
  Gi 2 : uav_library/UAV/Total applied moment/Moments 4 motors/Gi 1
  Gi 3 : uav_library/UAV/Total applied moment/Moments 4 motors/Gi 1
  Gi 4 : uav_library/UAV/Total applied moment/Moments 4 motors/Gi 1
  Math Function2 : Math  Operator=square  SaturateOnIntegerOverflow=on
  Product1 : Product
  Product2 : Product
  cross(PPi,Fi) 1 : Subsystem
  cross(PPi,Fi) 2 : uav_library/UAV/Total applied moment/Moments 4 motors/cross(PPi,Fi) 1
  cross(PPi,Fi) 3 : uav_library/UAV/Total applied moment/Moments 4 motors/cross(PPi,Fi) 1
  cross(PPi,Fi) 4 : uav_library/UAV/Total applied moment/Moments 4 motors/cross(PPi,Fi) 1
  Mb : Outport
  wires:
  [omegaDot] -> Product2/2
  [omega] -> Math Function2/1
  Math Function2/1 -> Product1/2
  Constant1/1 -> Product1/1
  Product1/1 -> Add/1
  Constant2/1 -> Product2/1
  Product2/1 -> Add/2
  Add/1 -> [taui]
  [sumGeneratedMoment] -> Add1/1
  [sumInducedMoment] -> Add1/2
  [sumGyroscopicMoment] -> Add1/3
  Add1/1 -> Mb/1
  Fi/1 -> [Fi]
  omega/1 -> [omega]
  omegaDot/1 -> [omegaDot]
  omegabt/1 -> [omegabt]
  Add2/1 -> [sumGeneratedMoment]
  Add3/1 -> [sumGyroscopicMoment]
  Add4/1 -> [sumInducedMoment]
  Constant8/1 -> cross(PPi,Fi) 1/1(PP)
  Constant6/1 -> cross(PPi,Fi) 1/2(iMotor)
  [Fi] -> cross(PPi,Fi) 1/3(Fi)
  cross(PPi,Fi) 1/1(cross(PPi,Fi)) -> Add2/1
  Constant17/1 -> cross(PPi,Fi) 2/1
  Constant9/1 -> cross(PPi,Fi) 2/2
  [Fi] -> cross(PPi,Fi) 2/3
  Constant11/1 -> cross(PPi,Fi) 3/1
  Constant10/1 -> cross(PPi,Fi) 3/2
  [Fi] -> cross(PPi,Fi) 3/3
  Constant14/1 -> cross(PPi,Fi) 4/1
  Constant13/1 -> cross(PPi,Fi) 4/2
  [Fi] -> cross(PPi,Fi) 4/3
  cross(PPi,Fi) 2/1 -> Add2/2
  cross(PPi,Fi) 3/1 -> Add2/3
  cross(PPi,Fi) 4/1 -> Add2/4
  Constant16/1 -> (-1)^iMotor taui 1/1(iMotor)
  [taui] -> (-1)^iMotor taui 1/2(taui)
  (-1)^iMotor taui 1/1((-1)^iMotor taui) -> Add4/1
  Constant3/1 -> (-1)^iMotor taui 2/1
  [taui] -> (-1)^iMotor taui 2/2
  Constant4/1 -> (-1)^iMotor taui 3/1
  [taui] -> (-1)^iMotor taui 3/2
  Constant12/1 -> (-1)^iMotor taui 4/1
  [taui] -> (-1)^iMotor taui 4/2
  (-1)^iMotor taui 2/1 -> Add4/2
  (-1)^iMotor taui 3/1 -> Add4/3
  (-1)^iMotor taui 4/1 -> Add4/4
  Constant27/1 -> Gi 1/1(iMotor)
  [omegabt] -> Gi 1/2(omegabt)
  [omega] -> Gi 1/3(omega)
  Gi 1/1(Gi) -> Add3/1
  Constant5/1 -> Gi 2/1
  [omegabt] -> Gi 2/2
  [omega] -> Gi 2/3
  Constant7/1 -> Gi 3/1
  [omegabt] -> Gi 3/2
  [omega] -> Gi 3/3
  Constant15/1 -> Gi 4/1
  [omegabt] -> Gi 4/2
  [omega] -> Gi 4/3
  Gi 2/1 -> Add3/2
  Gi 3/1 -> Add3/3
  Gi 4/1 -> Add3/4

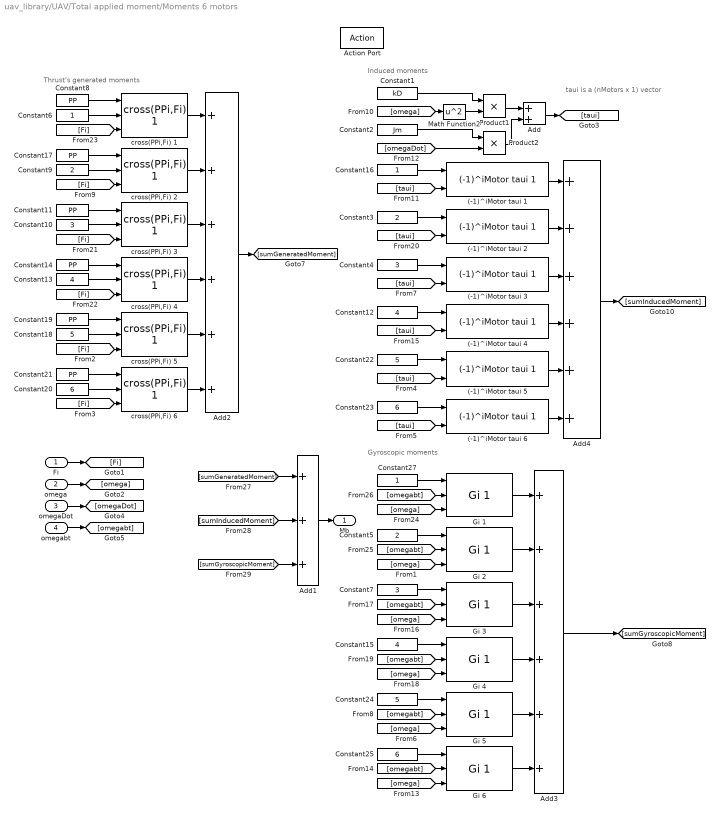
== system uav_library/UAV/Total applied moment/Moments 6 motors ==
  note: taui is a (nMotors x 1) vector
  note: Induced moments
  note: Gyroscopic moments
  note: Thrust's generated moments
  Fi : Inport
  omega : Inport  Port=2
  omegaDot : Inport  Port=3
  omegabt : Inport  Port=4
  Action Port : ActionPort  ActionType=elseif
  (-1)^iMotor taui {1..6} (6 alike) : uav_library/UAV/Total applied moment/Moments 4 motors/(-1)^iMotor taui 1
  Add : Sum
  Add1 : Sum  Inputs=+++
  Add2 : Sum  Inputs=++++++
  Add3 : Sum  Inputs=++++++
  Add4 : Sum  Inputs=++++++
  Constant1 : Constant  Value=kD
  Constant10 : Constant  Value=3
  Constant{8,11,14,17,19,21} (6 alike) : Constant  Value=PP
  Constant12 : Constant  Value=4
  Constant13 : Constant  Value=4
  Constant15 : Constant  Value=4
  Constant16 : Constant
  Constant18 : Constant  Value=5
  Constant2 : Constant  Value=Jm
  Constant20 : Constant  Value=6
  Constant22 : Constant  Value=5
  Constant23 : Constant  Value=6
  Constant24 : Constant  Value=5
  Constant25 : Constant  Value=6
  Constant27 : Constant
  Constant3 : Constant  Value=2
  Constant4 : Constant  Value=3
  Constant5 : Constant  Value=2
  Constant6 : Constant
  Constant7 : Constant  Value=3
  Constant9 : Constant  Value=2
  Gi {1..6} (6 alike) : uav_library/UAV/Total applied moment/Moments 4 motors/Gi 1
  Math Function2 : Math  Operator=square  SaturateOnIntegerOverflow=on
  Product1 : Product
  Product2 : Product
  cross(PPi,Fi) {1..6} (6 alike) : uav_library/UAV/Total applied moment/Moments 4 motors/cross(PPi,Fi) 1
  Mb : Outport
  wires:
  [omegaDot] -> Product2/2
  [omega] -> Math Function2/1
  Math Function2/1 -> Product1/2
  Constant1/1 -> Product1/1
  Product1/1 -> Add/1
  Constant2/1 -> Product2/1
  Product2/1 -> Add/2
  Add/1 -> [taui]
  [sumGeneratedMoment] -> Add1/1
  [sumInducedMoment] -> Add1/2
  [sumGyroscopicMoment] -> Add1/3
  Add1/1 -> Mb/1
  Fi/1 -> [Fi]
  omega/1 -> [omega]
  omegaDot/1 -> [omegaDot]
  omegabt/1 -> [omegabt]
  Add2/1 -> [sumGeneratedMoment]
  Add3/1 -> [sumGyroscopicMoment]
  Add4/1 -> [sumInducedMoment]
  Constant8/1 -> cross(PPi,Fi) 1/1
  Constant6/1 -> cross(PPi,Fi) 1/2
  [Fi] -> cross(PPi,Fi) 1/3
  cross(PPi,Fi) 1/1 -> Add2/1
  Constant17/1 -> cross(PPi,Fi) 2/1
  Constant9/1 -> cross(PPi,Fi) 2/2
  [Fi] -> cross(PPi,Fi) 2/3
  Constant11/1 -> cross(PPi,Fi) 3/1
  Constant10/1 -> cross(PPi,Fi) 3/2
  [Fi] -> cross(PPi,Fi) 3/3
  Constant14/1 -> cross(PPi,Fi) 4/1
  Constant13/1 -> cross(PPi,Fi) 4/2
  [Fi] -> cross(PPi,Fi) 4/3
  cross(PPi,Fi) 2/1 -> Add2/2
  cross(PPi,Fi) 3/1 -> Add2/3
  cross(PPi,Fi) 4/1 -> Add2/4
  Constant16/1 -> (-1)^iMotor taui 1/1
  [taui] -> (-1)^iMotor taui 1/2
  (-1)^iMotor taui 1/1 -> Add4/1
  Constant3/1 -> (-1)^iMotor taui 2/1
  [taui] -> (-1)^iMotor taui 2/2
  Constant4/1 -> (-1)^iMotor taui 3/1
  [taui] -> (-1)^iMotor taui 3/2
  Constant12/1 -> (-1)^iMotor taui 4/1
  [taui] -> (-1)^iMotor taui 4/2
  (-1)^iMotor taui 2/1 -> Add4/2
  (-1)^iMotor taui 3/1 -> Add4/3
  (-1)^iMotor taui 4/1 -> Add4/4
  Constant27/1 -> Gi 1/1
  [omegabt] -> Gi 1/2
  [omega] -> Gi 1/3
  Gi 1/1 -> Add3/1
  Constant5/1 -> Gi 2/1
  [omegabt] -> Gi 2/2
  [omega] -> Gi 2/3
  Constant7/1 -> Gi 3/1
  [omegabt] -> Gi 3/2
  [omega] -> Gi 3/3
  Constant15/1 -> Gi 4/1
  [omegabt] -> Gi 4/2
  [omega] -> Gi 4/3
  Gi 2/1 -> Add3/2
  Gi 3/1 -> Add3/3
  Gi 4/1 -> Add3/4
  Constant19/1 -> cross(PPi,Fi) 5/1
  Constant18/1 -> cross(PPi,Fi) 5/2
  [Fi] -> cross(PPi,Fi) 5/3
  Constant21/1 -> cross(PPi,Fi) 6/1
  Constant20/1 -> cross(PPi,Fi) 6/2
  [Fi] -> cross(PPi,Fi) 6/3
  cross(PPi,Fi) 5/1 -> Add2/5
  cross(PPi,Fi) 6/1 -> Add2/6
  Constant22/1 -> (-1)^iMotor taui 5/1
  [taui] -> (-1)^iMotor taui 5/2
  Constant23/1 -> (-1)^iMotor taui 6/1
  [taui] -> (-1)^iMotor taui 6/2
  (-1)^iMotor taui 6/1 -> Add4/6
  (-1)^iMotor taui 5/1 -> Add4/5
  Constant24/1 -> Gi 5/1
  [omegabt] -> Gi 5/2
  [omega] -> Gi 5/3
  Gi 5/1 -> Add3/5
  Constant25/1 -> Gi 6/1
  [omegabt] -> Gi 6/2
  [omega] -> Gi 6/3
  Gi 6/1 -> Add3/6

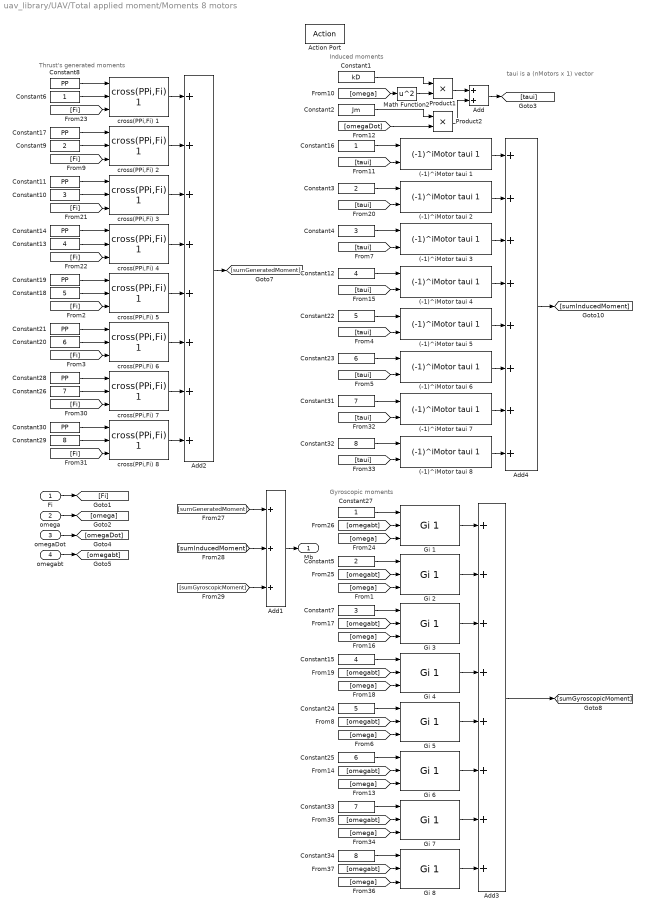
== system uav_library/UAV/Total applied moment/Moments 8 motors ==
  note: taui is a (nMotors x 1) vector
  note: Induced moments
  note: Gyroscopic moments
  note: Thrust's generated moments
  Fi : Inport
  omega : Inport  Port=2
  omegaDot : Inport  Port=3
  omegabt : Inport  Port=4
  Action Port : ActionPort  ActionType=elseif
  (-1)^iMotor taui {1..8} (8 alike) : uav_library/UAV/Total applied moment/Moments 4 motors/(-1)^iMotor taui 1
  Add : Sum
  Add1 : Sum  Inputs=+++
  Add2 : Sum  Inputs=++++++++
  Add3 : Sum  Inputs=++++++++
  Add4 : Sum  Inputs=++++++++
  Constant1 : Constant  Value=kD
  Constant10 : Constant  Value=3
  Constant{8,11,14,17,19,21,28,30} (8 alike) : Constant  Value=PP
  Constant12 : Constant  Value=4
  Constant13 : Constant  Value=4
  Constant15 : Constant  Value=4
  Constant16 : Constant
  Constant18 : Constant  Value=5
  Constant2 : Constant  Value=Jm
  Constant20 : Constant  Value=6
  Constant22 : Constant  Value=5
  Constant23 : Constant  Value=6
  Constant24 : Constant  Value=5
  Constant25 : Constant  Value=6
  Constant26 : Constant  Value=7
  Constant27 : Constant
  Constant29 : Constant  Value=8
  Constant3 : Constant  Value=2
  Constant31 : Constant  Value=7
  Constant32 : Constant  Value=8
  Constant33 : Constant  Value=7
  Constant34 : Constant  Value=8
  Constant4 : Constant  Value=3
  Constant5 : Constant  Value=2
  Constant6 : Constant
  Constant7 : Constant  Value=3
  Constant9 : Constant  Value=2
  Gi {1..8} (8 alike) : uav_library/UAV/Total applied moment/Moments 4 motors/Gi 1
  Math Function2 : Math  Operator=square  SaturateOnIntegerOverflow=on
  Product1 : Product
  Product2 : Product
  cross(PPi,Fi) {1..8} (8 alike) : uav_library/UAV/Total applied moment/Moments 4 motors/cross(PPi,Fi) 1
  Mb : Outport
  wires:
  [omegaDot] -> Product2/2
  [omega] -> Math Function2/1
  Math Function2/1 -> Product1/2
  Constant1/1 -> Product1/1
  Product1/1 -> Add/1
  Constant2/1 -> Product2/1
  Product2/1 -> Add/2
  Add/1 -> [taui]
  [sumGeneratedMoment] -> Add1/1
  [sumInducedMoment] -> Add1/2
  [sumGyroscopicMoment] -> Add1/3
  Add1/1 -> Mb/1
  Fi/1 -> [Fi]
  omega/1 -> [omega]
  omegaDot/1 -> [omegaDot]
  omegabt/1 -> [omegabt]
  Add2/1 -> [sumGeneratedMoment]
  Add3/1 -> [sumGyroscopicMoment]
  Add4/1 -> [sumInducedMoment]
  Constant8/1 -> cross(PPi,Fi) 1/1
  Constant6/1 -> cross(PPi,Fi) 1/2
  [Fi] -> cross(PPi,Fi) 1/3
  cross(PPi,Fi) 1/1 -> Add2/1
  Constant17/1 -> cross(PPi,Fi) 2/1
  Constant9/1 -> cross(PPi,Fi) 2/2
  [Fi] -> cross(PPi,Fi) 2/3
  Constant11/1 -> cross(PPi,Fi) 3/1
  Constant10/1 -> cross(PPi,Fi) 3/2
  [Fi] -> cross(PPi,Fi) 3/3
  Constant14/1 -> cross(PPi,Fi) 4/1
  Constant13/1 -> cross(PPi,Fi) 4/2
  [Fi] -> cross(PPi,Fi) 4/3
  cross(PPi,Fi) 2/1 -> Add2/2
  cross(PPi,Fi) 3/1 -> Add2/3
  cross(PPi,Fi) 4/1 -> Add2/4
  Constant16/1 -> (-1)^iMotor taui 1/1
  [taui] -> (-1)^iMotor taui 1/2
  (-1)^iMotor taui 1/1 -> Add4/1
  Constant3/1 -> (-1)^iMotor taui 2/1
  [taui] -> (-1)^iMotor taui 2/2
  Constant4/1 -> (-1)^iMotor taui 3/1
  [taui] -> (-1)^iMotor taui 3/2
  Constant12/1 -> (-1)^iMotor taui 4/1
  [taui] -> (-1)^iMotor taui 4/2
  (-1)^iMotor taui 2/1 -> Add4/2
  (-1)^iMotor taui 3/1 -> Add4/3
  (-1)^iMotor taui 4/1 -> Add4/4
  Constant27/1 -> Gi 1/1
  [omegabt] -> Gi 1/2
  [omega] -> Gi 1/3
  Gi 1/1 -> Add3/1
  Constant5/1 -> Gi 2/1
  [omegabt] -> Gi 2/2
  [omega] -> Gi 2/3
  Constant7/1 -> Gi 3/1
  [omegabt] -> Gi 3/2
  [omega] -> Gi 3/3
  Constant15/1 -> Gi 4/1
  [omegabt] -> Gi 4/2
  [omega] -> Gi 4/3
  Gi 2/1 -> Add3/2
  Gi 3/1 -> Add3/3
  Gi 4/1 -> Add3/4
  Constant19/1 -> cross(PPi,Fi) 5/1
  Constant18/1 -> cross(PPi,Fi) 5/2
  [Fi] -> cross(PPi,Fi) 5/3
  Constant21/1 -> cross(PPi,Fi) 6/1
  Constant20/1 -> cross(PPi,Fi) 6/2
  [Fi] -> cross(PPi,Fi) 6/3
  cross(PPi,Fi) 5/1 -> Add2/5
  cross(PPi,Fi) 6/1 -> Add2/6
  Constant22/1 -> (-1)^iMotor taui 5/1
  [taui] -> (-1)^iMotor taui 5/2
  Constant23/1 -> (-1)^iMotor taui 6/1
  [taui] -> (-1)^iMotor taui 6/2
  (-1)^iMotor taui 6/1 -> Add4/6
  (-1)^iMotor taui 5/1 -> Add4/5
  Constant24/1 -> Gi 5/1
  [omegabt] -> Gi 5/2
  [omega] -> Gi 5/3
  Gi 5/1 -> Add3/5
  Constant25/1 -> Gi 6/1
  [omegabt] -> Gi 6/2
  [omega] -> Gi 6/3
  Gi 6/1 -> Add3/6
  Constant28/1 -> cross(PPi,Fi) 7/1
  Constant26/1 -> cross(PPi,Fi) 7/2
  [Fi] -> cross(PPi,Fi) 7/3
  Constant30/1 -> cross(PPi,Fi) 8/1
  Constant29/1 -> cross(PPi,Fi) 8/2
  [Fi] -> cross(PPi,Fi) 8/3
  cross(PPi,Fi) 7/1 -> Add2/7
  cross(PPi,Fi) 8/1 -> Add2/8
  Constant31/1 -> (-1)^iMotor taui 7/1
  [taui] -> (-1)^iMotor taui 7/2
  Constant32/1 -> (-1)^iMotor taui 8/1
  [taui] -> (-1)^iMotor taui 8/2
  (-1)^iMotor taui 7/1 -> Add4/7
  (-1)^iMotor taui 8/1 -> Add4/8
  Constant33/1 -> Gi 7/1
  [omegabt] -> Gi 7/2
  [omega] -> Gi 7/3
  Constant34/1 -> Gi 8/1
  [omegabt] -> Gi 8/2
  [omega] -> Gi 8/3
  Gi 7/1 -> Add3/7
  Gi 8/1 -> Add3/8

== system uav_library/UAV/6DOF Euler/Body rate initial condition/Triggered Subsystem2 ==
  In1 : Inport
  Trigger : TriggerPort  TriggerType=falling  VariantControl=Variant
  Out1 : Outport
  wires:
  In1/1 -> Out1/1

== system uav_library/UAV/6DOF Euler/Body velocity initial condition/Triggered Subsystem2 ==
  In1 : Inport
  Trigger : TriggerPort  TriggerType=falling  VariantControl=Variant
  Out1 : Outport
  wires:
  In1/1 -> Out1/1

== system uav_library/UAV/6DOF Euler/Euleur angles initial condition/Triggered Subsystem2 ==
  In1 : Inport
  Trigger : TriggerPort  TriggerType=falling  VariantControl=Variant
  Out1 : Outport
  wires:
  In1/1 -> Out1/1

== system uav_library/UAV/6DOF Euler/Position initial condition/Triggered Subsystem2 ==
  In1 : Inport
  Trigger : TriggerPort  TriggerType=falling  VariantControl=Variant
  Out1 : Outport
  wires:
  In1/1 -> Out1/1

== system uav_library/UAV/DC Motors/DC Motor current dynamic w// La/ia initial condition ==
  Clock1 : Clock
  Constant3 : Constant  Value=iaInitial
  Constant6 : Constant  Value=iaDelay
  Sum4 : Sum  Inputs=|-+
  Triggered Subsystem2 : Subsystem  TreatAsAtomicUnit=on
  Out1 : Outport
  Out2 : Outport  Port=2
  wires:
  Constant6/1 -> Sum4/2
  Triggered Subsystem2/1(Out1) -> Out2/1
  Sum4/1 -> Out1/1, Triggered Subsystem2/Trigger
  Clock1/1 -> Sum4/1
  Constant3/1 -> Triggered Subsystem2/1(In1)

== system uav_library/UAV/DC Motors/omega initial condition/Triggered Subsystem2 ==
  In1 : Inport
  Trigger : TriggerPort  TriggerType=falling  VariantControl=Variant
  Out1 : Outport
  wires:
  In1/1 -> Out1/1

== system uav_library/UAV/Total applied moment/Moments 4 motors/(-1)^iMotor taui 1 ==
  iMotor : Inport
  taui : Inport  Port=2
  Add : Sum  Inputs=+-
  Constant1 : Constant  Value=0
  Constant2 : Constant  Value=-1
  Constant3 : Constant
  MATLAB Function1 : MATLAB Function  TreatAsAtomicUnit=on
  Math Function2 : Math  Operator=pow  SaturateOnIntegerOverflow=on
  Product1 : Product
  Vector Concatenate2 : Concatenate  NumInputs=3
  (-1)^iMotor taui : Outport
  wires:
  Vector Concatenate2/1 -> (-1)^iMotor taui/1
  MATLAB Function1/1(vectorOut) -> Product1/2
  Constant2/1 -> Math Function2/1
  taui/1 -> MATLAB Function1/1(matrixIn)
  iMotor/1 -> MATLAB Function1/2(rowIndex), Add/1
  Product1/1 -> Vector Concatenate2/3
  Math Function2/1 -> Product1/1
  Constant1/1 -> Vector Concatenate2/1, Vector Concatenate2/2
  Add/1 -> Math Function2/2
  Constant3/1 -> Add/2

== system uav_library/UAV/Total applied moment/Moments 4 motors/Gi 1 ==
  iMotor : Inport
  omegabt : Inport  Port=2
  omega : Inport  Port=3
  3x3 Cross Product1 : aerolibutil/3x3 Cross Product
  Constant3 : Constant  Value=-1
  Constant5 : Constant  Value=0
  MATLAB Function3 : MATLAB Function  TreatAsAtomicUnit=on
  Math Function : Math  Operator=pow  SaturateOnIntegerOverflow=on
  Product : Product
  Vector Concatenate1 : Concatenate  NumInputs=3
  Gi : Outport
  wires:
  omega/1 -> MATLAB Function3/1(matrixIn)
  Constant5/1 -> Vector Concatenate1/1, Vector Concatenate1/2
  Math Function/1 -> Product/1
  iMotor/1 -> Math Function/2, MATLAB Function3/2(rowIndex)
  Product/1 -> Vector Concatenate1/3
  omegabt/1 -> 3x3 Cross Product1/2
  3x3 Cross Product1/1 -> Gi/1
  MATLAB Function3/1(vectorOut) -> Product/2
  Vector Concatenate1/1 -> 3x3 Cross Product1/1
  Constant3/1 -> Math Function/1

== system uav_library/UAV/Total applied moment/Moments 4 motors/cross(PPi,Fi) 1 ==
  PP : Inport
  iMotor : Inport  Port=2
  Fi : Inport  Port=3
  3x3 Cross Product : aerolibutil/3x3 Cross Product
  Constant7 : Constant  Value=0
  MATLAB Function : MATLAB Function  TreatAsAtomicUnit=on
  MATLAB Function2 : MATLAB Function  TreatAsAtomicUnit=on
  Vector Concatenate3 : Concatenate  NumInputs=3
  cross(PPi,Fi) : Outport
  wires:
  Vector Concatenate3/1 -> 3x3 Cross Product/2
  Constant7/1 -> Vector Concatenate3/2, Vector Concatenate3/1
  3x3 Cross Product/1 -> cross(PPi,Fi)/1
  Fi/1 -> MATLAB Function2/1(matrixIn)
  MATLAB Function2/1(vectorOut) -> Vector Concatenate3/3
  MATLAB Function/1(vectorOut) -> 3x3 Cross Product/1
  PP/1 -> MATLAB Function/1(matrixIn)
  iMotor/1 -> MATLAB Function/2(colIndex), MATLAB Function2/2(rowIndex)

== system uav_library/UAV/DC Motors/DC Motor current dynamic w// La/ia initial condition/Triggered Subsystem2 ==
  In1 : Inport
  Trigger : TriggerPort  TriggerType=falling  VariantControl=Variant
  Out1 : Outport
  wires:
  In1/1 -> Out1/1

== matlab function uav_library/UAV/Total applied moment/Moments 4 motors/cross(PPi,Fi) 1/MATLAB Function ==
  data: matrixIn input; vectorOut output; colIndex input
function vectorOut  = extract_column(matrixIn,colIndex)
%#codegen

vectorOut = matrixIn(:,colIndex);

== matlab function uav_library/UAV/Total applied moment/Moments 4 motors/cross(PPi,Fi) 1/MATLAB Function2 ==
  data: matrixIn input; vectorOut output; rowIndex input
function vectorOut  = extract_row(matrixIn,rowIndex)
%#codegen

vectorOut = matrixIn(rowIndex,:);

== matlab function uav_library/UAV/Total applied moment/Moments 4 motors/(-1)^iMotor taui 1/MATLAB Function1 ==
  data: matrixIn input; vectorOut output; rowIndex input
function vectorOut  = extract_row(matrixIn,rowIndex)
%#codegen

vectorOut = matrixIn(rowIndex,:);

== matlab function uav_library/UAV/Total applied moment/Moments 4 motors/Gi 1/MATLAB Function3 ==
  data: matrixIn input; vectorOut output; rowIndex input
function vectorOut  = extract_row(matrixIn,rowIndex)
%#codegen

vectorOut = matrixIn(rowIndex,:);
